simulink model "receiveforce"  (R2014a)
settings: Solver=ode3  StartTime=0.0  StopTime=inf  FixedStep=0.001  RelTol=1e-3
undefined symbols (not defined in the file or in its folder): qualisys, ws
libraries: rtai_devices x1, sfbc_lib x1, rtai_utilities x1
settings Model: Creator=wirnshofer  LastModifiedBy=wirnshofer
settings DataIOCC: SignalLoggingSaveFormat=ModelDataLogs
settings RTWCC: SystemTargetFile=prt.tlc  TemplateMakefile=prt.tmf  Description=Linux PREEMPT_RT Real-Time Target  ProcessScript=prt_make_rtw_hook
settings STFCustomTargetCC: TargetLangStandard=C99 (ISO)  CodeReplacementLibrary=GNU C99 extensions  ModelReferenceCompliant=off  ConcurrentExecutionCompliant=off  MatFileLogging=on  SystemTargetFile=prt.tlc
settings GRTTargetCC: TargetLangStandard=C99 (ISO)  CodeReplacementLibrary=GNU C99 extensions  ModelReferenceCompliant=off  ParMdlRefBuildCompliant=off  CompOptLevelCompliant=off  ConcurrentExecutionCompliant=off  CombineOutputUpdateFcns=off  CPPClassGenCompliant=off  GRTInterface=on

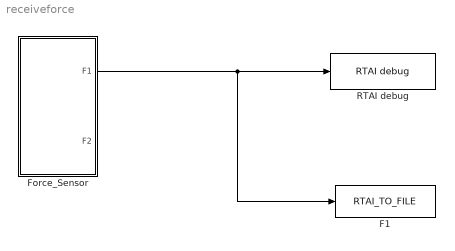
== system receiveforce ==
  F1 : rtai_devices/RTAI_TO_FILE  N=3  InType=double  FileName='F1.dat'  FpOutStr='%f '  TStartStop=[1.1 10]  T=0.001  Confirm=off  Cutoff=off
  Force_Sensor : Subsystem
  RTAI debug : rtai_utilities/RTAI debug  rate=1
  wires:
  Force_Sensor/1(F1) -> F1/1, RTAI debug/1

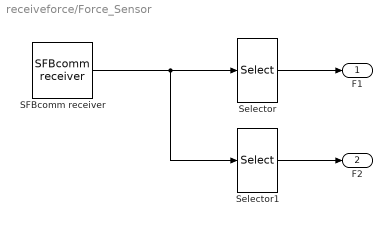
== system receiveforce/Force_Sensor ==
  SFBcomm receiver : sfbc_lib/SFBcomm receiver  localPort=33001  streamID=1  remoteSettings=qualisys-ws:11112  portNames=A  portWidths=6  outputLatency=off  outputIdleTime=off  connectTimeout=200  sampleTime=-1
  Selector : Selector  InputPortWidth=6  Indices=1:3
  Selector1 : Selector  InputPortWidth=6  Indices=4:6
  F1 : Outport
  F2 : Outport  Port=2
  wires:
  SFBcomm receiver/1 -> Selector1/1, Selector/1
  Selector/1 -> F1/1
  Selector1/1 -> F2/1
